simulink model "HDLLTE"  (R2017b)
settings: Solver=FixedStepDiscrete  StartTime=0.0  StopTime=simParams.stopTime  RelTol=1e-3
InitFcn:
  | simParams = hdlcoder_lteofdm_modDetectref_init;
  | simParams = hdlcoder_lteofdm_modDetecthdl_init(simParams);
StopFcn:
  | hdlcoder_lteofdm_modDetect_analyze;
undefined symbols (not defined in the file): fft_size
libraries: hdlsllib x29, simulink x22, simulink_need_slupdate x13, dspxfrm3 x2, commchan3 x1, dspmlti4 x1, commrflib2 x1, hdlcodermisc x1, dspsigops x1, dspmathops x1, dspsrcs4 x1
(part 3 of 3)

== system HDLLTE/LTE_Detector_HDL/PSS_Detection/Peak_Detection/Local_Search_PSS0/maximum ==
  note: After 10 clock cycles, output
      | maximum value and corresponding
      | index value
  note: Hold index value (out of 10)
      | for current maximum value
  note: Count to 10
  note: Check for new maximum value
  dataIn : Inport
  Enb : Inport  Port=2
  Constant : Constant  Value=10  VectorParams1D=off  OutDataTypeStr=fixdt(0,4,0)  SampleTime=simParams.TsRx
  Constant1 : Constant  Value=0  VectorParams1D=off  OutDataTypeStr=fixdt(0,22,20)  SampleTime=simParams.TsRx
  Delay Reset : Subsystem
  Delay Reset2 : Subsystem
  HDL Counter : hdlsllib/Sources/HDL Counter  CountType=Count limited  CountInit=1  CountStep=1  CountMax=10  CountFromType=Initial value  CountFrom=1  CountResetPort=on  CountLoadPort=off  CountEnbPort=on  CountDirPort=off  CountDataType=Unsigned  CountWordLen=4  CountFracLen=0  CountSampTime=1
      settings: SourceProductBaseCode=HD
  Logical Operator1 : Logic  Operator=NOT  IconShape=distinctive  AllPortsSameDT=off  OutDataTypeStr=boolean
  Relational Operator1 : RelationalOperator  Operator=>  OutDataTypeStr=boolean  RndMeth=Nearest
  Relational Operator2 : RelationalOperator  Operator===  OutDataTypeStr=boolean  RndMeth=Nearest
  Switch : Switch  Criteria=u2 > Threshold
  Switch1 : Switch  Criteria=u2 > Threshold
  MaxVal : Outport  InitialOutput=0
  MaxIdx : Outport  Port=2  InitialOutput=0
  wires:
  Relational Operator1/1 -> Delay Reset2/2(E), Delay Reset/2(E)
  Delay Reset/1(y) -> Switch/1, Relational Operator1/2
  Enb/1 -> Logical Operator1/1, HDL Counter/2
  dataIn/1 -> Delay Reset/1(u), Relational Operator1/1
  Constant/1 -> Relational Operator2/2
  Switch/1 -> MaxVal/1
  Relational Operator2/1 -> Switch/2, Switch1/2
  Constant1/1 -> Switch/3, Switch1/3
  Switch1/1 -> MaxIdx/1
  Delay Reset2/1(y) -> Switch1/1
  Logical Operator1/1 -> HDL Counter/1, Delay Reset2/3(R), Delay Reset/3(R)
  HDL Counter/1 -> Delay Reset2/1(u), Relational Operator2/1

== system HDLLTE/LTE_Detector_HDL/PSS_Detection/Peak_Detection/Local_Search_PSS1/maximum ==
  note: Check for new maximum value
  note: Count to 10
  note: Hold index value (out of 10)
      | for current maximum value
  note: After 10 clock cycles, output
      | maximum value and corresponding
      | index value
  dataIn : Inport
  Enb : Inport  Port=2
  Constant : Constant  Value=10  VectorParams1D=off  OutDataTypeStr=fixdt(0,4,0)  SampleTime=simParams.TsRx
  Constant1 : Constant  Value=0  VectorParams1D=off  OutDataTypeStr=fixdt(0,22,20)  SampleTime=simParams.TsRx
  Delay Reset : Subsystem
  Delay Reset2 : Subsystem
  HDL Counter : hdlsllib/Sources/HDL Counter  CountType=Count limited  CountInit=1  CountStep=1  CountMax=10  CountFromType=Initial value  CountFrom=1  CountResetPort=on  CountLoadPort=off  CountEnbPort=on  CountDirPort=off  CountDataType=Unsigned  CountWordLen=4  CountFracLen=0  CountSampTime=1
      settings: SourceProductBaseCode=HD
  Logical Operator1 : Logic  Operator=NOT  IconShape=distinctive  AllPortsSameDT=off  OutDataTypeStr=boolean
  Relational Operator1 : RelationalOperator  Operator=>  OutDataTypeStr=boolean  RndMeth=Nearest
  Relational Operator2 : RelationalOperator  Operator===  OutDataTypeStr=boolean  RndMeth=Nearest
  Switch : Switch  Criteria=u2 > Threshold
  Switch1 : Switch  Criteria=u2 > Threshold
  MaxVal : Outport  InitialOutput=0
  MaxIdx : Outport  Port=2  InitialOutput=0
  wires:
  HDL Counter/1 -> Relational Operator2/1, Delay Reset2/1(u)
  Logical Operator1/1 -> Delay Reset/3(R), Delay Reset2/3(R), HDL Counter/1
  Delay Reset2/1(y) -> Switch1/1
  Switch1/1 -> MaxIdx/1
  Constant1/1 -> Switch1/3, Switch/3
  Relational Operator2/1 -> Switch1/2, Switch/2
  Switch/1 -> MaxVal/1
  Constant/1 -> Relational Operator2/2
  dataIn/1 -> Relational Operator1/1, Delay Reset/1(u)
  Enb/1 -> HDL Counter/2, Logical Operator1/1
  Delay Reset/1(y) -> Relational Operator1/2, Switch/1
  Relational Operator1/1 -> Delay Reset/2(E), Delay Reset2/2(E)

== system HDLLTE/LTE_Detector_HDL/PSS_Detection/Peak_Detection/Local_Search_PSS2/maximum ==
  note: After 10 clock cycles, output
      | maximum value and corresponding
      | index value
  note: Hold index value (out of 10)
      | for current maximum value
  note: Count to 10
  note: Check for new maximum value
  dataIn : Inport
  Enb : Inport  Port=2
  Constant : Constant  Value=10  VectorParams1D=off  OutDataTypeStr=fixdt(0,4,0)  SampleTime=simParams.TsRx
  Constant1 : Constant  Value=0  VectorParams1D=off  OutDataTypeStr=fixdt(0,22,20)  SampleTime=simParams.TsRx
  Delay Reset : Subsystem
  Delay Reset2 : Subsystem
  HDL Counter : hdlsllib/Sources/HDL Counter  CountType=Count limited  CountInit=1  CountStep=1  CountMax=10  CountFromType=Initial value  CountFrom=1  CountResetPort=on  CountLoadPort=off  CountEnbPort=on  CountDirPort=off  CountDataType=Unsigned  CountWordLen=4  CountFracLen=0  CountSampTime=1
      settings: SourceProductBaseCode=HD
  Logical Operator1 : Logic  Operator=NOT  IconShape=distinctive  AllPortsSameDT=off  OutDataTypeStr=boolean
  Relational Operator1 : RelationalOperator  Operator=>  OutDataTypeStr=boolean  RndMeth=Nearest
  Relational Operator2 : RelationalOperator  Operator===  OutDataTypeStr=boolean  RndMeth=Nearest
  Switch : Switch  Criteria=u2 > Threshold
  Switch1 : Switch  Criteria=u2 > Threshold
  MaxVal : Outport  InitialOutput=0
  MaxIdx : Outport  Port=2  InitialOutput=0
  wires:
  Relational Operator1/1 -> Delay Reset2/2(E), Delay Reset/2(E)
  Delay Reset/1(y) -> Switch/1, Relational Operator1/2
  Enb/1 -> Logical Operator1/1, HDL Counter/2
  dataIn/1 -> Delay Reset/1(u), Relational Operator1/1
  Constant/1 -> Relational Operator2/2
  Switch/1 -> MaxVal/1
  Relational Operator2/1 -> Switch/2, Switch1/2
  Constant1/1 -> Switch/3, Switch1/3
  Switch1/1 -> MaxIdx/1
  Delay Reset2/1(y) -> Switch1/1
  Logical Operator1/1 -> HDL Counter/1, Delay Reset2/3(R), Delay Reset/3(R)
  HDL Counter/1 -> Delay Reset2/1(u), Relational Operator2/1

== system HDLLTE/LTE_Detector_HDL/SSS_Detection/SSS_Dot_Product/Delay Reset/Reset Delay ==
  note: Reset
  u1 : Inport
  R1 : Inport  Port=2
  FixPt Constant : Constant  DisableCoverage=on  Value=0  OutDataTypeStr=uint8  SampleTime=simParams.TsRx
  FixPt Logical Operator : Logic  DisableCoverage=on  Operator=OR  AllPortsSameDT=off  OutDataTypeStr=fixdt(0, 8)
  FixPt Unit Delay1 : UnitDelay  DisableCoverage=on  SampleTime=-1  HasFrameUpgradeWarning=off
  FixPt Unit Delay2 : UnitDelay  DisableCoverage=on  InitialCondition=1  SampleTime=-1
  Init : Switch  Criteria=u2 > Threshold  OutDataTypeStr=Inherit: Inherit via back propagation  ZeroCross=off
  Initial Condition : Constant  DisableCoverage=on  Value=complex(0)  OutDataTypeStr=Inherit: Inherit via back propagation  SampleTime=simParams.TsRx
  Reset : Switch  Criteria=u2 > Threshold  OutDataTypeStr=Inherit: Inherit via back propagation  ZeroCross=off
  Out1 : Outport
  wires:
  Reset/1 -> FixPt Unit Delay1/1  "Xnew"
  Init/1 -> Out1/1
  R1/1 -> Reset/2, FixPt Logical Operator/1
  FixPt Logical Operator/1 -> Init/2
  FixPt Unit Delay2/1 -> FixPt Logical Operator/2
  FixPt Constant/1 -> FixPt Unit Delay2/1
  Initial Condition/1 -> Reset/1, Init/1  "Initial Value"
  FixPt Unit Delay1/1 -> Init/3  "Xold"
  u1/1 -> Reset/3

== system HDLLTE/LTE_Detector_HDL/PSS_Detection/Peak_Detection/Local_Search_PSS0/maximum/Delay Reset ==
  note: Enable
  u : Inport
  E : Inport  Port=2
  R : Inport  Port=3
  Enable : Switch  Criteria=u2 > Threshold  OutDataTypeStr=Inherit: Inherit via back propagation  ZeroCross=off
  Reset Delay : Subsystem
  y : Outport
  wires:
  E/1 -> Enable/2
  Reset Delay/1(Out1) -> Enable/3, y/1
  u/1 -> Enable/1
  Enable/1 -> Reset Delay/1(u1)
  R/1 -> Reset Delay/2(R1)

== system HDLLTE/LTE_Detector_HDL/PSS_Detection/Peak_Detection/Local_Search_PSS0/maximum/Delay Reset2 ==
  note: Enable
  u : Inport
  E : Inport  Port=2
  R : Inport  Port=3
  Enable : Switch  Criteria=u2 > Threshold  OutDataTypeStr=Inherit: Inherit via back propagation  ZeroCross=off
  Reset Delay : Subsystem
  y : Outport
  wires:
  E/1 -> Enable/2
  Reset Delay/1(Out1) -> Enable/3, y/1
  u/1 -> Enable/1
  Enable/1 -> Reset Delay/1(u1)
  R/1 -> Reset Delay/2(R1)

== system HDLLTE/LTE_Detector_HDL/PSS_Detection/Peak_Detection/Local_Search_PSS1/maximum/Delay Reset ==
  note: Enable
  u : Inport
  E : Inport  Port=2
  R : Inport  Port=3
  Enable : Switch  Criteria=u2 > Threshold  OutDataTypeStr=Inherit: Inherit via back propagation  ZeroCross=off
  Reset Delay : Subsystem
  y : Outport
  wires:
  R/1 -> Reset Delay/2(R1)
  Enable/1 -> Reset Delay/1(u1)
  u/1 -> Enable/1
  Reset Delay/1(Out1) -> y/1, Enable/3
  E/1 -> Enable/2

== system HDLLTE/LTE_Detector_HDL/PSS_Detection/Peak_Detection/Local_Search_PSS1/maximum/Delay Reset2 ==
  note: Enable
  u : Inport
  E : Inport  Port=2
  R : Inport  Port=3
  Enable : Switch  Criteria=u2 > Threshold  OutDataTypeStr=Inherit: Inherit via back propagation  ZeroCross=off
  Reset Delay : Subsystem
  y : Outport
  wires:
  R/1 -> Reset Delay/2(R1)
  Enable/1 -> Reset Delay/1(u1)
  u/1 -> Enable/1
  Reset Delay/1(Out1) -> y/1, Enable/3
  E/1 -> Enable/2

== system HDLLTE/LTE_Detector_HDL/PSS_Detection/Peak_Detection/Local_Search_PSS2/maximum/Delay Reset ==
  note: Enable
  u : Inport
  E : Inport  Port=2
  R : Inport  Port=3
  Enable : Switch  Criteria=u2 > Threshold  OutDataTypeStr=Inherit: Inherit via back propagation  ZeroCross=off
  Reset Delay : Subsystem
  y : Outport
  wires:
  E/1 -> Enable/2
  Reset Delay/1(Out1) -> Enable/3, y/1
  u/1 -> Enable/1
  Enable/1 -> Reset Delay/1(u1)
  R/1 -> Reset Delay/2(R1)

== system HDLLTE/LTE_Detector_HDL/PSS_Detection/Peak_Detection/Local_Search_PSS2/maximum/Delay Reset2 ==
  note: Enable
  u : Inport
  E : Inport  Port=2
  R : Inport  Port=3
  Enable : Switch  Criteria=u2 > Threshold  OutDataTypeStr=Inherit: Inherit via back propagation  ZeroCross=off
  Reset Delay : Subsystem
  y : Outport
  wires:
  E/1 -> Enable/2
  Reset Delay/1(Out1) -> Enable/3, y/1
  u/1 -> Enable/1
  Enable/1 -> Reset Delay/1(u1)
  R/1 -> Reset Delay/2(R1)

== system HDLLTE/LTE_Detector_HDL/PSS_Detection/Peak_Detection/Local_Search_PSS0/maximum/Delay Reset/Reset Delay ==
  note: Reset
  u1 : Inport
  R1 : Inport  Port=2
  FixPt Constant : Constant  DisableCoverage=on  Value=0  OutDataTypeStr=fixdt(0,8,0)  SampleTime=simParams.TsRx
  FixPt Logical Operator : Logic  DisableCoverage=on  Operator=OR  AllPortsSameDT=off  OutDataTypeStr=fixdt(0, 8)
  FixPt Unit Delay1 : UnitDelay  DisableCoverage=on  SampleTime=-1  HasFrameUpgradeWarning=off
  FixPt Unit Delay2 : UnitDelay  DisableCoverage=on  InitialCondition=1  SampleTime=-1
  Init : Switch  Criteria=u2 > Threshold  OutDataTypeStr=Inherit: Inherit via back propagation  ZeroCross=off
  Initial Condition : Constant  DisableCoverage=on  Value=0  OutDataTypeStr=Inherit: Inherit via back propagation  SampleTime=simParams.TsRx
  Reset : Switch  Criteria=u2 > Threshold  OutDataTypeStr=Inherit: Inherit via back propagation  ZeroCross=off
  Out1 : Outport
  wires:
  u1/1 -> Reset/3
  FixPt Unit Delay1/1 -> Init/3  "Xold"
  Initial Condition/1 -> Init/1, Reset/1  "Initial Value"
  FixPt Constant/1 -> FixPt Unit Delay2/1
  FixPt Unit Delay2/1 -> FixPt Logical Operator/2
  FixPt Logical Operator/1 -> Init/2
  R1/1 -> FixPt Logical Operator/1, Reset/2
  Init/1 -> Out1/1
  Reset/1 -> FixPt Unit Delay1/1  "Xnew"

== system HDLLTE/LTE_Detector_HDL/PSS_Detection/Peak_Detection/Local_Search_PSS0/maximum/Delay Reset2/Reset Delay ==
  note: Reset
  u1 : Inport
  R1 : Inport  Port=2
  FixPt Constant : Constant  DisableCoverage=on  Value=0  OutDataTypeStr=fixdt(0,8,0)  SampleTime=simParams.TsRx
  FixPt Logical Operator : Logic  DisableCoverage=on  Operator=OR  AllPortsSameDT=off  OutDataTypeStr=fixdt(0, 8)
  FixPt Unit Delay1 : UnitDelay  DisableCoverage=on  SampleTime=-1  HasFrameUpgradeWarning=off
  FixPt Unit Delay2 : UnitDelay  DisableCoverage=on  InitialCondition=1  SampleTime=-1
  Init : Switch  Criteria=u2 > Threshold  OutDataTypeStr=Inherit: Inherit via back propagation  ZeroCross=off
  Initial Condition : Constant  DisableCoverage=on  Value=0  OutDataTypeStr=Inherit: Inherit via back propagation  SampleTime=simParams.TsRx
  Reset : Switch  Criteria=u2 > Threshold  OutDataTypeStr=Inherit: Inherit via back propagation  ZeroCross=off
  Out1 : Outport
  wires:
  u1/1 -> Reset/3
  FixPt Unit Delay1/1 -> Init/3  "Xold"
  Initial Condition/1 -> Init/1, Reset/1  "Initial Value"
  FixPt Constant/1 -> FixPt Unit Delay2/1
  FixPt Unit Delay2/1 -> FixPt Logical Operator/2
  FixPt Logical Operator/1 -> Init/2
  R1/1 -> FixPt Logical Operator/1, Reset/2
  Init/1 -> Out1/1
  Reset/1 -> FixPt Unit Delay1/1  "Xnew"

== system HDLLTE/LTE_Detector_HDL/PSS_Detection/Peak_Detection/Local_Search_PSS1/maximum/Delay Reset/Reset Delay ==
  note: Reset
  u1 : Inport
  R1 : Inport  Port=2
  FixPt Constant : Constant  DisableCoverage=on  Value=0  OutDataTypeStr=fixdt(0,8,0)  SampleTime=simParams.TsRx
  FixPt Logical Operator : Logic  DisableCoverage=on  Operator=OR  AllPortsSameDT=off  OutDataTypeStr=fixdt(0, 8)
  FixPt Unit Delay1 : UnitDelay  DisableCoverage=on  SampleTime=-1  HasFrameUpgradeWarning=off
  FixPt Unit Delay2 : UnitDelay  DisableCoverage=on  InitialCondition=1  SampleTime=-1
  Init : Switch  Criteria=u2 > Threshold  OutDataTypeStr=Inherit: Inherit via back propagation  ZeroCross=off
  Initial Condition : Constant  DisableCoverage=on  Value=0  OutDataTypeStr=Inherit: Inherit via back propagation  SampleTime=simParams.TsRx
  Reset : Switch  Criteria=u2 > Threshold  OutDataTypeStr=Inherit: Inherit via back propagation  ZeroCross=off
  Out1 : Outport
  wires:
  Reset/1 -> FixPt Unit Delay1/1  "Xnew"
  Init/1 -> Out1/1
  R1/1 -> Reset/2, FixPt Logical Operator/1
  FixPt Logical Operator/1 -> Init/2
  FixPt Unit Delay2/1 -> FixPt Logical Operator/2
  FixPt Constant/1 -> FixPt Unit Delay2/1
  Initial Condition/1 -> Reset/1, Init/1  "Initial Value"
  FixPt Unit Delay1/1 -> Init/3  "Xold"
  u1/1 -> Reset/3

== system HDLLTE/LTE_Detector_HDL/PSS_Detection/Peak_Detection/Local_Search_PSS1/maximum/Delay Reset2/Reset Delay ==
  note: Reset
  u1 : Inport
  R1 : Inport  Port=2
  FixPt Constant : Constant  DisableCoverage=on  Value=0  OutDataTypeStr=fixdt(0,8,0)  SampleTime=simParams.TsRx
  FixPt Logical Operator : Logic  DisableCoverage=on  Operator=OR  AllPortsSameDT=off  OutDataTypeStr=fixdt(0, 8)
  FixPt Unit Delay1 : UnitDelay  DisableCoverage=on  SampleTime=-1  HasFrameUpgradeWarning=off
  FixPt Unit Delay2 : UnitDelay  DisableCoverage=on  InitialCondition=1  SampleTime=-1
  Init : Switch  Criteria=u2 > Threshold  OutDataTypeStr=Inherit: Inherit via back propagation  ZeroCross=off
  Initial Condition : Constant  DisableCoverage=on  Value=0  OutDataTypeStr=Inherit: Inherit via back propagation  SampleTime=simParams.TsRx
  Reset : Switch  Criteria=u2 > Threshold  OutDataTypeStr=Inherit: Inherit via back propagation  ZeroCross=off
  Out1 : Outport
  wires:
  Reset/1 -> FixPt Unit Delay1/1  "Xnew"
  Init/1 -> Out1/1
  R1/1 -> Reset/2, FixPt Logical Operator/1
  FixPt Logical Operator/1 -> Init/2
  FixPt Unit Delay2/1 -> FixPt Logical Operator/2
  FixPt Constant/1 -> FixPt Unit Delay2/1
  Initial Condition/1 -> Reset/1, Init/1  "Initial Value"
  FixPt Unit Delay1/1 -> Init/3  "Xold"
  u1/1 -> Reset/3

== system HDLLTE/LTE_Detector_HDL/PSS_Detection/Peak_Detection/Local_Search_PSS2/maximum/Delay Reset/Reset Delay ==
  note: Reset
  u1 : Inport
  R1 : Inport  Port=2
  FixPt Constant : Constant  DisableCoverage=on  Value=0  OutDataTypeStr=fixdt(0,8,0)  SampleTime=simParams.TsRx
  FixPt Logical Operator : Logic  DisableCoverage=on  Operator=OR  AllPortsSameDT=off  OutDataTypeStr=fixdt(0, 8)
  FixPt Unit Delay1 : UnitDelay  DisableCoverage=on  SampleTime=-1  HasFrameUpgradeWarning=off
  FixPt Unit Delay2 : UnitDelay  DisableCoverage=on  InitialCondition=1  SampleTime=-1
  Init : Switch  Criteria=u2 > Threshold  OutDataTypeStr=Inherit: Inherit via back propagation  ZeroCross=off
  Initial Condition : Constant  DisableCoverage=on  Value=0  OutDataTypeStr=Inherit: Inherit via back propagation  SampleTime=simParams.TsRx
  Reset : Switch  Criteria=u2 > Threshold  OutDataTypeStr=Inherit: Inherit via back propagation  ZeroCross=off
  Out1 : Outport
  wires:
  u1/1 -> Reset/3
  FixPt Unit Delay1/1 -> Init/3  "Xold"
  Initial Condition/1 -> Init/1, Reset/1  "Initial Value"
  FixPt Constant/1 -> FixPt Unit Delay2/1
  FixPt Unit Delay2/1 -> FixPt Logical Operator/2
  FixPt Logical Operator/1 -> Init/2
  R1/1 -> FixPt Logical Operator/1, Reset/2
  Init/1 -> Out1/1
  Reset/1 -> FixPt Unit Delay1/1  "Xnew"

== system HDLLTE/LTE_Detector_HDL/PSS_Detection/Peak_Detection/Local_Search_PSS2/maximum/Delay Reset2/Reset Delay ==
  note: Reset
  u1 : Inport
  R1 : Inport  Port=2
  FixPt Constant : Constant  DisableCoverage=on  Value=0  OutDataTypeStr=fixdt(0,8,0)  SampleTime=simParams.TsRx
  FixPt Logical Operator : Logic  DisableCoverage=on  Operator=OR  AllPortsSameDT=off  OutDataTypeStr=fixdt(0, 8)
  FixPt Unit Delay1 : UnitDelay  DisableCoverage=on  SampleTime=-1  HasFrameUpgradeWarning=off
  FixPt Unit Delay2 : UnitDelay  DisableCoverage=on  InitialCondition=1  SampleTime=-1
  Init : Switch  Criteria=u2 > Threshold  OutDataTypeStr=Inherit: Inherit via back propagation  ZeroCross=off
  Initial Condition : Constant  DisableCoverage=on  Value=0  OutDataTypeStr=Inherit: Inherit via back propagation  SampleTime=simParams.TsRx
  Reset : Switch  Criteria=u2 > Threshold  OutDataTypeStr=Inherit: Inherit via back propagation  ZeroCross=off
  Out1 : Outport
  wires:
  u1/1 -> Reset/3
  FixPt Unit Delay1/1 -> Init/3  "Xold"
  Initial Condition/1 -> Init/1, Reset/1  "Initial Value"
  FixPt Constant/1 -> FixPt Unit Delay2/1
  FixPt Unit Delay2/1 -> FixPt Logical Operator/2
  FixPt Logical Operator/1 -> Init/2
  R1/1 -> FixPt Logical Operator/1, Reset/2
  Init/1 -> Out1/1
  Reset/1 -> FixPt Unit Delay1/1  "Xnew"

== matlab function HDLLTE/LTE_Modulator_HDL/CP_Extension_Windowing/symbolRAM read controller ==
  settings: fimath=hdlfimath
  data: WRITE_COUNTER input; read_address output; countValid output; read_valid output; nFFT input; FFT_size_minus_CP input; windowing input
function [read_address, countValid, read_valid] = read_addr_control(WRITE_COUNTER,nFFT,FFT_size_minus_CP, windowing)
%#codegen

persistent READ_COUNTER;

if isempty(READ_COUNTER)
    READ_COUNTER=uint16(nFFT*2-1);
end

read_address=READ_COUNTER;

% Data is valid if CP is being passed through (WRITE_COUNTER >= FFT_size_minus_CP)
% OR IFFT frame is currently being read from RAM (READ_COUNTER<nFFT)
read_valid=(uint16(WRITE_COUNTER)>=uint16(FFT_size_minus_CP)) || (READ_COUNTER<uint16(nFFT));

if uint16(WRITE_COUNTER) < uint16(FFT_size_minus_CP)
    countValid = (WRITE_COUNTER>=uint16(FFT_size_minus_CP)-uint16(windowing)-uint16(1)) || (READ_COUNTER<uint16(nFFT));
else
    countValid = read_valid;
end


if WRITE_COUNTER==uint16(nFFT-1)
    % Reset WRITE_COUNTER to zero if count reaches nFFT-windowing-1
    READ_COUNTER=uint16(0);
else
    % While READ_COUNTER is less than nFFT
    if READ_COUNTER<uint16(nFFT)
        % Increment READ_COUNTER
        READ_COUNTER=READ_COUNTER+uint16(1);
    end
end

== matlab function HDLLTE/LTE_Detector_HDL/PSS_Detection/Determine_Primary_Cell_ID/PipelinedMax ==
  data: x input; val output; idx output uint16
function [val,idx] = PipelinedMax(x)
    % Returns the maximum value in the vector x. x must be of length 3.
    % This requires two comparisons. To optimized for HDL timing performance,
    % a single register is placed between the two comparisons.
    %#codegen
    
    persistent valReg;    % max value out of 1 and 2
    persistent idxReg;    % zero based index
    
    if isempty(valReg)
        valReg = cast(0,'like',x(1));
        idxReg = uint16(0);
    end
    
    % second comparison, reads registers before they are written to
    if valReg > x(3)
        val = valReg;
        idx = idxReg;
    else
        val = x(3);
        idx = uint16(2);
    end
    
    % first comparison, writes to registers
    if x(1) > x(2)
        valReg(:) = x(1);
        idxReg(:) = uint16(0);
    else
        valReg(:) = x(2);
        idxReg(:) = uint16(1);
    end
    
end

== matlab function HDLLTE/LTE_Modulator_HDL/CP_Extension_Windowing/Check Window Multiply  ==
  data: Sample_Index input; nFFT input; pass_through output; FFT_size_minus_CP input; cp_win_index output
function [pass_through, cp_win_index]=check_pass(Sample_Index,nFFT,FFT_size_minus_CP)
%#codegen
pass_through=false; cp_win_index = uint16(0);
if (uint16(Sample_Index)>=FFT_size_minus_CP) && (uint16(Sample_Index)<=uint16(nFFT))
  pass_through=true;
  cp_win_index = uint16(Sample_Index) - uint16(FFT_size_minus_CP);
end

== matlab function HDLLTE/LTE_Modulator_HDL/CP_Extension_Windowing/Check Window Add and Passthrough ==
  data: Sample_Index input; nFFT input; pass_through output; FFT_size_minus_CP input; add_window output; windowing input uint16
function [pass_through, add_window] =check_pass(Sample_Index,nFFT,FFT_size_minus_CP, windowing)
%#codegen
pass_through=false; add_window = false;
if (uint16(Sample_Index)>=uint16(FFT_size_minus_CP)) && (uint16(Sample_Index)<=uint16(nFFT))
  pass_through=true;
end

if (uint16(Sample_Index)>=uint16(FFT_size_minus_CP)-uint16(windowing)) && (uint16(Sample_Index)<=uint16(nFFT))
    add_window = true;
end
